simulink model "Likitha_Version_3_1"  (R2025b)
settings: Solver=VariableStepAuto  StartTime=0.0  StopTime=0.3  RelTol=1e-3
undefined symbols (not defined in the file): Ion, Lithium
libraries: spsBatteryLib x50, spsSeriesRLCBranchLib x15, spsCurrentMeasurementLib x10, spsVoltageMeasurementLib x10, spsIdealSwitchLib x9, spsMosfetLib x7, slpidlib x4, spsPWMGeneratorDCDCLib x2, spspowerguiLib x2, spsACVoltageSourceLib x1, eeHysteresisControl x1, spsDCMachineLib x1
(part 3 of 3)

== system Likitha_Version_3_1/Subsystem11/6 ==
  Battery1 : spsBatteryLib/Battery  BatType=Lithium-Ion  NomV=3.3  NomQ=2.7  SOC=97.5  Batt_Tr=30  PresetModel=on  MaxQ=2.7  MinV=2.475  FullV=3.8412  Dis_rate=1.1739  R=0.012222  Normal_OP=2.4417  expZone="[3.5653     0.13265]"
  Bus Selector : BusSelector  OutputSignals=SOC (%),Current (A),Voltage (V)
  Product : Product
  Scope : Scope  NumInputPorts=4
      settings: ActiveDisplayYMinimum=99.92989  ActiveDisplayYMaximum=100.00779
  + : PMIOPort  Side=Right
  - : PMIOPort  Port=2  Side=Right
  tag scope: cm_6=global, soc6=global, vm_6=global
  wires:
  Battery1/1 -> Bus Selector/1
  Bus Selector/1 -> [soc6], Scope/1  "<SOC (%)>"
  Product/1 -> Scope/4
  Bus Selector/2 -> [cm_6], Product/1, Scope/2  "<Current (A)>"
  Bus Selector/3 -> [vm_6], Scope/3, Product/2  "<Voltage (V)>"
  connections:
  +/RConn1 -- Battery1/LConn1
  -/RConn1 -- Battery1/LConn2

== system Likitha_Version_3_1/Subsystem11/7 ==
  Battery1 : spsBatteryLib/Battery  BatType=Lithium-Ion  NomV=3.3  NomQ=2.7  SOC=97  Batt_Tr=30  PresetModel=on  MaxQ=2.7  MinV=2.475  FullV=3.8412  Dis_rate=1.1739  R=0.012222  Normal_OP=2.4417  expZone="[3.5653     0.13265]"
  Bus Selector : BusSelector  OutputSignals=SOC (%),Current (A),Voltage (V)
  Product : Product
  Scope : Scope  NumInputPorts=4
      settings: ActiveDisplayYMinimum=99.92989  ActiveDisplayYMaximum=100.00779
  + : PMIOPort  Side=Right
  - : PMIOPort  Port=2  Side=Right
  tag scope: cm_7=global, soc7=global, vm_7=global
  wires:
  Battery1/1 -> Bus Selector/1
  Bus Selector/1 -> [soc7], Scope/1  "<SOC (%)>"
  Product/1 -> Scope/4
  Bus Selector/2 -> [cm_7], Product/1, Scope/2  "<Current (A)>"
  Bus Selector/3 -> [vm_7], Scope/3, Product/2  "<Voltage (V)>"
  connections:
  +/RConn1 -- Battery1/LConn1
  -/RConn1 -- Battery1/LConn2

== system Likitha_Version_3_1/Subsystem11/8 ==
  Battery1 : spsBatteryLib/Battery  BatType=Lithium-Ion  NomV=3.3  NomQ=2.7  SOC=96.5  Batt_Tr=30  PresetModel=on  MaxQ=2.7  MinV=2.475  FullV=3.8412  Dis_rate=1.1739  R=0.012222  Normal_OP=2.4417  expZone="[3.5653     0.13265]"
  Bus Selector : BusSelector  OutputSignals=SOC (%),Current (A),Voltage (V)
  Product : Product
  Scope : Scope  NumInputPorts=4
      settings: ActiveDisplayYMinimum=99.92989  ActiveDisplayYMaximum=100.00779
  + : PMIOPort  Side=Right
  - : PMIOPort  Port=2  Side=Right
  tag scope: cm_8=global, soc8=global, vm_8=global
  wires:
  Battery1/1 -> Bus Selector/1
  Bus Selector/1 -> [soc8], Scope/1  "<SOC (%)>"
  Product/1 -> Scope/4
  Bus Selector/2 -> [cm_8], Product/1, Scope/2  "<Current (A)>"
  Bus Selector/3 -> Scope/3, [vm_8], Product/2  "<Voltage (V)>"
  connections:
  +/RConn1 -- Battery1/LConn1
  -/RConn1 -- Battery1/LConn2

== system Likitha_Version_3_1/Subsystem11/9 ==
  Battery1 : spsBatteryLib/Battery  BatType=Lithium-Ion  NomV=3.3  NomQ=2.7  SOC=96  Batt_Tr=30  PresetModel=on  MaxQ=2.7  MinV=2.475  FullV=3.8412  Dis_rate=1.1739  R=0.012222  Normal_OP=2.4417  expZone="[3.5653     0.13265]"
  Bus Selector : BusSelector  OutputSignals=SOC (%),Current (A),Voltage (V)
  Product : Product
  Scope : Scope  NumInputPorts=4
      settings: ActiveDisplayYMinimum=99.92989  ActiveDisplayYMaximum=100.00779
  + : PMIOPort  Side=Right
  - : PMIOPort  Port=2  Side=Right
  tag scope: cm_9=global, soc9=global, vm_9=global
  wires:
  Battery1/1 -> Bus Selector/1
  Bus Selector/1 -> [soc9], Scope/1  "<SOC (%)>"
  Product/1 -> Scope/4
  Bus Selector/2 -> [cm_9], Product/1, Scope/2  "<Current (A)>"
  Bus Selector/3 -> [vm_9], Scope/3, Product/2  "<Voltage (V)>"
  connections:
  +/RConn1 -- Battery1/LConn1
  -/RConn1 -- Battery1/LConn2

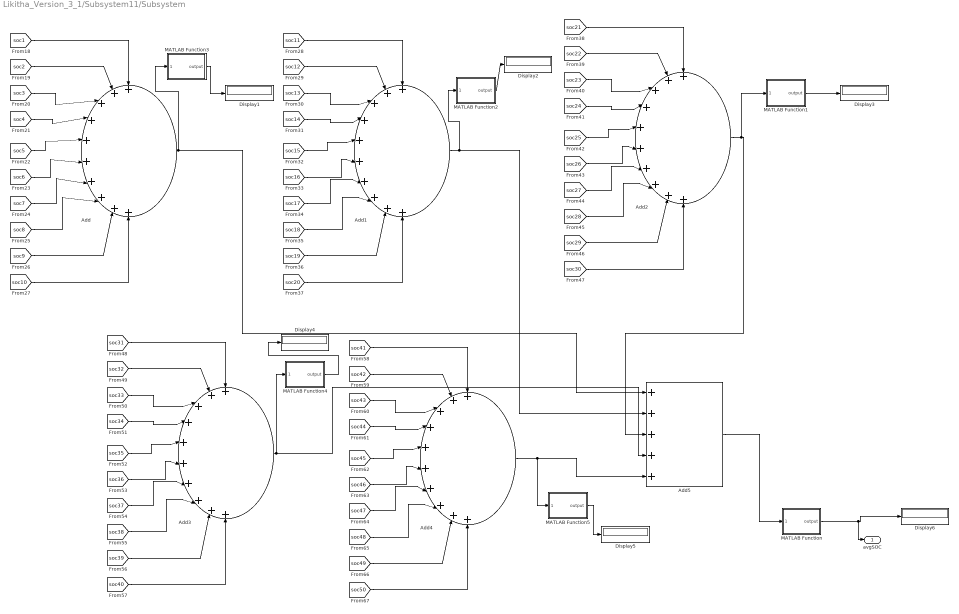
== system Likitha_Version_3_1/Subsystem11/Subsystem ==
  Add{,1..4} (5 alike) : Sum  Inputs=++++++++++
  Add5 : Sum  Inputs=+++++
  Display{1..6} (6 alike) : Display
  MATLAB Function : MATLAB Function  TreatAsAtomicUnit=on
  MATLAB Function1 : MATLAB Function  TreatAsAtomicUnit=on
  MATLAB Function2 : MATLAB Function  TreatAsAtomicUnit=on
  MATLAB Function3 : MATLAB Function  TreatAsAtomicUnit=on
  MATLAB Function4 : MATLAB Function  TreatAsAtomicUnit=on
  MATLAB Function5 : MATLAB Function  TreatAsAtomicUnit=on
  avgSOC : Outport
  wires:
  [soc16] -> Add1/6
  [soc31] -> Add3/1
  [soc42] -> Add4/2
  [soc6] -> Add/6
  Add3/1 -> MATLAB Function4/1(inputValue), Add5/4
  [soc33] -> Add3/3
  [soc12] -> Add1/2
  [soc50] -> Add4/10
  [soc1] -> Add/1
  [soc13] -> Add1/3
  [soc39] -> Add3/9
  Add2/1 -> MATLAB Function1/1(inputValue), Add5/3
  [soc28] -> Add2/8
  [soc3] -> Add/3
  [soc17] -> Add1/7
  [soc36] -> Add3/6
  [soc2] -> Add/2
  [soc45] -> Add4/5
  [soc49] -> Add4/9
  [soc27] -> Add2/7
  [soc48] -> Add4/8
  [soc15] -> Add1/5
  [soc20] -> Add1/10
  [soc43] -> Add4/3
  [soc26] -> Add2/6
  Add1/1 -> MATLAB Function2/1(inputValue), Add5/2
  [soc41] -> Add4/1
  [soc46] -> Add4/6
  [soc14] -> Add1/4
  [soc24] -> Add2/4
  [soc22] -> Add2/2
  [soc44] -> Add4/4
  [soc47] -> Add4/7
  [soc38] -> Add3/8
  [soc21] -> Add2/1
  [soc18] -> Add1/8
  [soc7] -> Add/7
  [soc19] -> Add1/9
  [soc9] -> Add/9
  [soc40] -> Add3/10
  [soc4] -> Add/4
  [soc11] -> Add1/1
  [soc35] -> Add3/5
  [soc8] -> Add/8
  Add/1 -> Add5/1, MATLAB Function3/1(inputValue)
  [soc5] -> Add/5
  [soc37] -> Add3/7
  [soc29] -> Add2/9
  Add4/1 -> MATLAB Function5/1(inputValue), Add5/5
  [soc34] -> Add3/4
  [soc32] -> Add3/2
  [soc10] -> Add/10
  [soc25] -> Add2/5
  [soc30] -> Add2/10
  [soc23] -> Add2/3
  Add5/1 -> MATLAB Function/1(inputValue)
  MATLAB Function/1(output) -> avgSOC/1, Display6/1
  MATLAB Function1/1(output) -> Display3/1
  MATLAB Function2/1(output) -> Display2/1
  MATLAB Function3/1(output) -> Display1/1
  MATLAB Function4/1(output) -> Display4/1
  MATLAB Function5/1(output) -> Display5/1

== system Likitha_Version_3_1/AC to DC/Subsystem1/Subsystem ==
  Iref : Inport
  Clock : Clock
  Constant : Constant  Value=2*pi/3
  Gain : Gain  Gain=2*pi*50
  Gain2 : Gain  Gain=2*pi*50
  Gain3 : Gain  Gain=2*pi*50
  Mux : Mux  Inputs=3
  Product : Product
  Sin : Trigonometry
  Sin1 : Trigonometry
  Sin2 : Trigonometry
  Subtract : Sum  Inputs=+-
  Subtract1 : Sum
  Out1 : Outport
  wires:
  Mux/1 -> Product/1
  Gain/1 -> Sin/1
  Sin2/1 -> Mux/3
  Clock/1 -> Gain3/1, Gain2/1, Gain/1
  Sin/1 -> Mux/1
  Constant/1 -> Subtract1/2, Subtract/2
  Subtract/1 -> Sin1/1
  Sin1/1 -> Mux/2
  Gain2/1 -> Subtract/1
  Gain3/1 -> Subtract1/1
  Subtract1/1 -> Sin2/1
  Product/1 -> Out1/1
  Iref/1 -> Product/2

== matlab function Likitha_Version_3_1/Subsystem2/MATLAB Function ==
  settings: updateMethod=DISCRETE  sampleTime=0.1
  data: SOC output; SOH output; SOP output; SOC_in input; DOD output; ROH output; Vp1 input; Vp2 input; R0_in input; RUL output; CycleCount output; AddParams output; Cap_in input; I_meas input; V_meas input; T_meas input; dt input
function [SOC, SOH, SOP, DOD, ROH, RUL, CycleCount, AddParams] = ParameterEstimator(...
    SOC_in, Vp1, Vp2, R0_in, Cap_in, I_meas, V_meas, T_meas, dt)
% ParameterEstimator - Computes all battery health and performance parameters
% 
% Inputs:
%   SOC_in   : Estimated SOC from filter (%)
%   Vp1, Vp2 : Polarization voltages (V)
%   R0_in    : Internal resistance (Ohm)
%   Cap_in   : Estimated capacity (Ah)
%   I_meas   : Measured current (A)
%   V_meas   : Measured voltage (V)
%   T_meas   : Measured temperature (°C)
%   dt       : Time step (s)
%
% Outputs:
%   SOC        : State of Charge (%) – passed through
%   SOH        : State of Health (%) – based on capacity fade
%   SOP        : State of Power (W) – max discharge power
%   DOD        : Depth of Discharge (%) = 100 - SOC
%   ROH        : Internal resistance (Ohm) – filtered version
%   RUL        : Remaining Useful Life (cycles)
%   CycleCount : Number of equivalent full cycles
%   AddParams  : [1x15] array of additional health indices:
%       1.  V_avg            : Average voltage (V)
%       2.  I_avg            : Average current (A)
%       3.  P_avg            : Average power (W)
%       4.  stress_idx       : Stress index (0-1)
%       5.  aging_rate_frac  : Aging rate (fraction per cycle)
%       6.  energy_kWh       : Cumulative energy throughput (kWh)
%       7.  degrad_idx       : Degradation index (1 - SOH/100)
%       8.  T_idx            : Temperature index (0-1, optimum 25°C)
%       9.  health_idx       : Overall health index (0-1)
%       10. I_peak           : Peak current (A, with decay)
%       11. V_min            : Minimum voltage (V, with recovery)
%       12. T_max            : Maximum temperature (°C, with decay)
%       13. Ah_charge_total  : Total charge Ampere-hours (Ah)
%       14. Ah_discharge_total: Total discharge Ampere-hours (Ah)
%       15. overtime_sec     : Cumulative time above 45°C (s)

% -------------------------------------------------------------------------
% Persistent variables for historical data
% -------------------------------------------------------------------------
persistent nominal_capacity cycleCount Ah_throughput lastSOC
persistent V_avg I_avg P_avg E_throughput I_peak V_min T_max
persistent Ah_charge Ah_discharge overtemp_time
persistent first_run

% -------------------------------------------------------------------------
% Initialization
% -------------------------------------------------------------------------
if isempty(first_run)
    nominal_capacity = 50;        % Nominal capacity at BOL (Ah)
    cycleCount = 0;
    Ah_throughput = 0;
    lastSOC = 100;
    
    V_avg = V_meas;
    I_avg = I_meas;
    P_avg = V_meas * I_meas;
    E_throughput = 0;
    I_peak = abs(I_meas);
    V_min = V_meas;
    T_max = T_meas;
    Ah_charge = 0;
    Ah_discharge = 0;
    overtemp_time = 0;
    
    first_run = true;
end

% -------------------------------------------------------------------------
% Basic passed-through parameters
% -------------------------------------------------------------------------
SOC = SOC_in;                       % %
DOD = 100 - SOC;                    % %
ROH = R0_in;                         % Ohm (could apply low-pass filter)
SOH = (Cap_in / nominal_capacity) * 100;   % %
SOH = max(0, min(100, SOH));

% -------------------------------------------------------------------------
% Cycle counting (full cycle when SOC crosses 20% -> 80%)
% -------------------------------------------------------------------------
if lastSOC <= 20 && SOC >= 80
    cycleCount = cycleCount + 1;
end
lastSOC = SOC;
CycleCount = cycleCount;

% -------------------------------------------------------------------------
% Update Ah throughput and energy throughput
% -------------------------------------------------------------------------
dAh = abs(I_meas) * dt / 3600;          % Ampere-hours
Ah_throughput = Ah_throughput + dAh;

dEnergy = abs(V_meas * I_meas) * dt / 3600 / 1000;   % kWh
E_throughput = E_throughput + dEnergy;

% Separate charge/discharge Ah
if I_meas < 0   % charging
    Ah_charge = Ah_charge + abs(I_meas) * dt / 3600;
elseif I_meas > 0
    Ah_discharge = Ah_discharge + I_meas * dt / 3600;
end

% -------------------------------------------------------------------------
% State of Power (SOP) estimation
% -------------------------------------------------------------------------
% Use OCV from SOC (simplified linear model – replace with lookup if available)
OCV = 0.04 * SOC + 3.0;   % V
Vmin = 2.7;   % Minimum allowed voltage
I_max_dis = (OCV - Vmin) / (ROH + 1e-6);   % A
SOP = I_max_dis * Vmin;   % W (max discharge power)

% -------------------------------------------------------------------------
% Remaining Useful Life (RUL) based on aging rate
% -------------------------------------------------------------------------
% Compute aging rate per cycle from capacity fade
if cycleCount > 0
    aging_rate_per_cycle = (100 - SOH) / cycleCount;   % % loss per cycle
else
    aging_rate_per_cycle = 0.01;   % default 0.01% per cycle
end
cycles_to_80 = (SOH - 80) / aging_rate_per_cycle;
RUL = max(0, cycles_to_80);

% -------------------------------------------------------------------------
% Additional 15 health parameters (exponential moving averages, peaks, etc.)
% -------------------------------------------------------------------------
alpha = 0.01;   % smoothing factor for averages (~100 samples time constant)

% 1. Average voltage
V_avg = (1 - alpha) * V_avg + alpha * V_meas;

% 2. Average current
I_avg = (1 - alpha) * I_avg + alpha * I_meas;

% 3. Average power
P_avg = (1 - alpha) * P_avg + alpha * (V_meas * I_meas);

% 4. Stress index (function of C-rate and temperature)
C_rate = abs(I_meas) / Cap_in;   % Current in C-rate
stress_idx = min(1, (C_rate / 2) * (T_meas / 50));

% 5. Aging rate (as fraction per cycle)
aging_rate_frac = aging_rate_per_cycle / 100;

% 6. Energy throughput (already computed in kWh)
energy_kWh = E_throughput;

% 7. Degradation index
degrad_idx = 1 - SOH/100;

% 8. Temperature index (normalized 0-1, optimum 25°C)
T_idx = max(0, min(1, 1 - abs(T_meas - 25)/50));

% 9. Overall health index (weighted combination)
health_idx = 0.5*(SOH/100) + 0.3*(1-stress_idx) + 0.2*T_idx;

% 10. Peak current (with slow decay)
I_peak = max(abs(I_meas), 0.999 * I_peak);

% 11. Minimum voltage (with slow recovery)
V_min = min(V_meas, V_min + 0.001);

% 12. Maximum temperature (with slow decay)
T_max = max(T_meas, T_max - 0.01);

% 13. Charge throughput (Ah)
Ah_charge_total = Ah_charge;

% 14. Discharge throughput (Ah)
Ah_discharge_total = Ah_discharge;

% 15. Time at over-temperature (cumulative seconds above 45°C)
if T_meas > 45
    overtemp_time = overtemp_time + dt;
end
overtime_sec = overtemp_time;

% Pack all additional parameters into a 1x15 array
AddParams = [V_avg, I_avg, P_avg, stress_idx, aging_rate_frac, ...
             energy_kWh, degrad_idx, T_idx, health_idx, I_peak, ...
             V_min, T_max, Ah_charge_total, Ah_discharge_total, overtime_sec];

% Ensure all outputs are real
SOC = real(SOC);
SOH = real(SOH);
SOP = real(SOP);
DOD = real(DOD);
ROH = real(ROH);
RUL = real(RUL);
CycleCount = real(CycleCount);
AddParams = real(AddParams);

end

== matlab function Likitha_Version_3_1/Subsystem11/Subsystem/MATLAB Function1 ==
  data: inputValue input; output output
function output = divideByFifty(inputValue)
% This function divides the input decimal value by 10

output = inputValue / 10;

end

== matlab function Likitha_Version_3_1/Subsystem11/Subsystem/MATLAB Function2 ==
  data: inputValue input; output output
function output = divideByFifty(inputValue)
% This function divides the input decimal value by 10

output = inputValue / 10;

end

== matlab function Likitha_Version_3_1/Subsystem11/Subsystem/MATLAB Function3 ==
  data: inputValue input; output output
function output = divideByFifty(inputValue)
% This function divides the input decimal value by 10

output = inputValue / 10;

end

== matlab function Likitha_Version_3_1/Subsystem11/Subsystem/MATLAB Function4 ==
  data: inputValue input; output output
function output = divideByFifty(inputValue)
% This function divides the input decimal value by 10

output = inputValue / 10;

end

== matlab function Likitha_Version_3_1/Subsystem11/Subsystem/MATLAB Function5 ==
  data: inputValue input; output output
function output = divideByFifty(inputValue)
% This function divides the input decimal value by 10

output = inputValue / 10;

end

== matlab function Likitha_Version_3_1/Controller/BMS ==
  settings: updateMethod=DISCRETE
  data: SOC input; C output; t input
function C = fcn_charge_discharge_time(SOC, t)
% C = 1 → Charge
% C = 0 → Discharge

%% USER SETTINGS
T_charge    = 100;   % Charge duration (sec)
T_discharge = 100;   % Discharge duration (sec)
MaxCycles   = 5;     % Number of cycles

%% Persistent variables
persistent last_value t_ref cycle mode
% mode: 1 = charge, 0 = discharge

if isempty(last_value)
    last_value = 1;      % Start with charging
    t_ref = t;
    cycle = 0;
    mode = 1;
end

%% Stop switching after max cycles
if cycle >= MaxCycles
    C = last_value;
    return;
end

%% Time-based switching
if mode == 1   % Charging
    if (t - t_ref) >= T_charge || SOC >= 80
        mode = 0;       % Switch to discharge
        t_ref = t;
    end
else           % Discharging
    if (t - t_ref) >= T_discharge || SOC <= 20
        mode = 1;       % Switch to charge
        t_ref = t;
        cycle = cycle + 1;  % Count full cycle
    end
end

%% Output
C = mode;
last_value = C;

end

== matlab function Likitha_Version_3_1/Subsystem11/Subsystem/MATLAB Function ==
  data: inputValue input; output output
function output = divideByFifty(inputValue)
% This function divides the input decimal value by 50

output = inputValue / 50;

end

== stateflow chart Likitha_Version_3_1/Charger/5SCCC ==
  state Initialize
    entry:
    signal=1;
    Iref=1*C;
  state fifth_stage
    entry:
    Iref=0.01*C;
  state end
    entry:
    signal=2;
  state back_to_charge
    entry:
    signal=1;
    Iref=0;
  state first_stage
    entry:
    Iref=0.32*C;
  state fourth_stage
    entry:
    Iref=0.057*C;
  state second_stage
    entry:
    Iref=0.1*C;
  state third_stage
    entry:
    Iref=0.1*C;
  back_to_charge -> (junction 27)
  (junction 27) -> end [order 2]
  (default) -> (junction 27)
  Initialize -> (junction 27) [order 2] : [sw==0]
  (junction 27) -> Initialize [order 1] : [sw==1]
  end -> back_to_charge : [sw==1]
  fifth_stage -> end [order 1] : [Vpeak<=Vb]
  first_stage -> Initialize [order 2] : [sw==0]
  fifth_stage -> fourth_stage [order 2] : [sw==0]
  Initialize -> first_stage [order 1] : [Vpeak<=Vb]
  fourth_stage -> fifth_stage [order 1] : [Vpeak<=Vb]
  fourth_stage -> third_stage [order 2] : [sw==0]
  second_stage -> first_stage [order 2] : [sw==0]
  first_stage -> second_stage [order 1] : [Vpeak<=Vb]
  third_stage -> fourth_stage [order 1] : [Vpeak<=Vb]
  second_stage -> third_stage [order 1] : [Vpeak<=Vb]
  third_stage -> second_stage [order 2] : [sw==0]
  data: Vpeak input; Vb input; Iref output; signal output; C input; sw input

== matlab function Likitha_Version_3_1/Subsystem11/MATLAB Function ==
  settings: updateMethod=DISCRETE
  data: V1 input; S1 output; V2 input; V3 input; V4 input; V5 input; S2 output; S3 output; S4 output; S5 output
function [S1,S2,S3,S4,S5] = battery_pack_switch_logic(V1,V2,V3,V4,V5)
% Outputs: 1 = ON, 0 = OFF

%% Parameters
V_over = 35;      % Over-voltage threshold
V_under = 30;     % Under-voltage threshold
V_tol = 0.5;      % Voltage balancing tolerance

V = [V1 V2 V3 V4 V5];

%% Persistent switch states (memory)
persistent S
if isempty(S)
    S = ones(1,5);   % All ON initially
end

%% Average voltage of active packs
V_active = V(S == 1);
if isempty(V_active)
    V_avg = mean(V);   % fallback
else
    V_avg = mean(V_active);
end

%% Control logic
for i = 1:5

    % Protection: Over / Under Voltage
    if V(i) > V_over || V(i) < V_under
        S(i) = 0;   % Force OFF
    end

    % Re-enable logic (balancing condition)
    if S(i) == 0
        if abs(V(i) - V_avg) <= V_tol
            S(i) = 1;   % Turn ON again
        end
    end

end

%% Outputs
S1 = S(1);
S2 = S(2);
S3 = S(3);
S4 = S(4);
S5 = S(5);

end

== matlab function Likitha_Version_3_1/Subsystem1/MATLAB Function ==
  settings: updateMethod=DISCRETE  sampleTime=0.1
  data: V_meas input; SOC_est output; I_meas input; T_meas input; dt input; Vp1_est output; Vp2_est output; R0_est output; Cap_est output; OCV_est output; Vfilt output
function [SOC_est, Vp1_est, Vp2_est, R0_est, Cap_est, OCV_est, Vfilt] = AEKF_Battery(V_meas, I_meas, T_meas, dt)
% AEKF_Battery - Adaptive Extended Kalman Filter for Li-ion battery state estimation
% 
% Implements a second-order RC model:
%   V_t = OCV(SOC) - I*R0 - Vp1 - Vp2 + v
%   d(Vp1)/dt = -Vp1/(R1*C1) + I/C1
%   d(Vp2)/dt = -Vp2/(R2*C2) + I/C2
%   d(SOC)/dt = -I / (3600*Cap)   (Cap in Ah)
%
% State vector: x = [SOC; Vp1; Vp2; bias; 1/Cap]  (bias compensates sensor offset)
% Outputs:
%   SOC_est, Vp1_est, Vp2_est, R0_est, Cap_est, OCV_est, Vfilt (filtered voltage)

% -------------------------------------------------------------------------
% Persistent variables (retained between calls)
% -------------------------------------------------------------------------
persistent x P Q R wk k dt_prev
persistent R0 R1 C1 R2 C2         % Model parameters (may depend on SOC/T)
persistent nominal_capacity        % Ah
persistent first_run

% -------------------------------------------------------------------------
% Initialization (tune these values to match your cell)
% -------------------------------------------------------------------------
if isempty(first_run)
    first_run = false;   % Will be set to true after init
    nominal_capacity = 50;   % Nominal capacity (Ah)
    
    % Initial state [SOC(%); Vp1(V); Vp2(V); bias(V); invCap(1/Ah)]
    x = [100; 0; 0; 0; 1/nominal_capacity];
    
    % Initial covariance
    P = diag([1, 0.1, 0.1, 0.01, 1e-6]);
    
    % Process noise covariance (will be adapted)
    Q = diag([0.01, 0.001, 0.001, 1e-6, 1e-8]);
    
    % Measurement noise variance (will be adapted)
    R = 0.1;   % Voltage measurement noise (V^2)
    
    % Fixed model parameters (you may replace with SOC/T lookup)
    R0 = 0.05;   % Ohm
    R1 = 0.02;   % Ohm
    C1 = 2000;   % Farad
    R2 = 0.03;   % Ohm
    C2 = 5000;   % Farad
    
    dt_prev = dt;
    wk = 0;      % Process noise scaling placeholder
end

% -------------------------------------------------------------------------
% Time constant checks (avoid division by zero)
% -------------------------------------------------------------------------
tau1 = max(R1*C1, 1e-6);
tau2 = max(R2*C2, 1e-6);

% -------------------------------------------------------------------------
% 1. Prediction step (a priori estimate)
% -------------------------------------------------------------------------
% Extract states
SOC = x(1);
Vp1 = x(2);
Vp2 = x(3);
bias = x(4);
invCap = x(5);
Cap = 1 / max(invCap, 1e-6);   % Capacity in Ah

% State transition function f(x,u)
%   SOC_{k+1} = SOC_k - (I * dt) / (3600 * Cap)
%   Vp1_{k+1} = exp(-dt/tau1)*Vp1_k + (1-exp(-dt/tau1))*R1*I
%   Vp2_{k+1} = exp(-dt/tau2)*Vp2_k + (1-exp(-dt/tau2))*R2*I
%   bias_{k+1} = bias_k
%   invCap_{k+1} = invCap_k   (slowly varying)

% Pre-compute exponentials
alpha1 = exp(-dt / tau1);
alpha2 = exp(-dt / tau2);

% Predicted states
x_pred = [SOC - (I_meas * dt) / (3600 * Cap);
          alpha1 * Vp1 + (1 - alpha1) * R1 * I_meas;
          alpha2 * Vp2 + (1 - alpha2) * R2 * I_meas;
          bias;
          invCap];

% State transition Jacobian F = df/dx
F = [1, 0, 0, 0,  (I_meas * dt) / (3600 * Cap^2);   % dSOC/dinvCap
     0, alpha1, 0, 0, 0;
     0, 0, alpha2, 0, 0;
     0, 0, 0, 1, 0;
     0, 0, 0, 0, 1];

% Predicted covariance
P_pred = F * P * F' + Q;

% -------------------------------------------------------------------------
% 2. OCV model (as function of SOC)
% -------------------------------------------------------------------------
% Replace with a lookup table for higher accuracy:
%   OCV = interp1(SOC_points, OCV_points, SOC, 'pchip');
% Here we use a 5th-order polynomial (example coefficients)
OCV = polyval([-1.5e-6, 2e-4, -0.01, 0.3, 0.1, 3.0], SOC);
dOCV_dSOC = polyval([-7.5e-6, 8e-4, -0.03, 0.6, 0.1], SOC);   % Derivative

% -------------------------------------------------------------------------
% 3. Measurement update (using voltage measurement)
% -------------------------------------------------------------------------
% Predicted terminal voltage
V_pred = OCV - I_meas * R0 - Vp1 - Vp2 + bias;

% Measurement Jacobian H = dV/dx
H = [dOCV_dSOC, -1, -1, 1, 0];   % Note: no direct dependence on invCap

% Innovation
y = V_meas - V_pred;

% Innovation covariance
S = H * P_pred * H' + R;

% Kalman gain
K = P_pred * H' / S;

% State update
x_upd = x_pred + K * y;

% Covariance update
P_upd = (eye(5) - K * H) * P_pred;

% -------------------------------------------------------------------------
% 4. Adaptive noise covariance estimation (simplified Sage-Husa)
% -------------------------------------------------------------------------
% Update measurement noise covariance R using residual smoothing
persistent r_sum r_count
if isempty(r_sum)
    r_sum = 0;
    r_count = 0;
end
r_sum = r_sum + y^2;
r_count = r_count + 1;
if r_count > 100
    R_est = r_sum / r_count;
    R = 0.95 * R + 0.05 * R_est;   % Smooth update
    r_sum = 0;
    r_count = 0;
end

% Process noise Q could also be adapted, but keep simple here

% -------------------------------------------------------------------------
% 5. Apply constraints and update persistent states
% -------------------------------------------------------------------------
x_upd(1) = max(0, min(100, x_upd(1)));   % SOC between 0-100%
x_upd(5) = max(1/(2*nominal_capacity), min(1/(0.5*nominal_capacity), x_upd(5))); % Capacity between 50% and 200% of nominal (optional)

x = x_upd;
P = P_upd;

% -------------------------------------------------------------------------
% Output assignments
% -------------------------------------------------------------------------
SOC_est = x(1);
Vp1_est = x(2);
Vp2_est = x(3);
bias_est = x(4);
Cap_est = 1 / x(5);
R0_est = R0;   % Could also be estimated online, but kept fixed here
OCV_est = OCV;
Vfilt = V_pred;   % Filtered voltage (same as prediction after update? Actually we can output filtered voltage)
% Alternatively, use updated states to compute a refined voltage:
Vfilt = OCV_est - I_meas * R0 - Vp1_est - Vp2_est + bias_est;

end
